simulink library "CTRL_LO_ST1_YAWTRQLATDIST"  (R2023b)
settings: Solver=VariableStepAuto  StartTime=0.0  StopTime=10.0  RelTol=1e-3
undefined symbols (not defined in the file): p_RadWhlDynFr_m, p_RadWhlDynRe_m
settings Model: Creator=blatak  LastModifiedBy=blatak

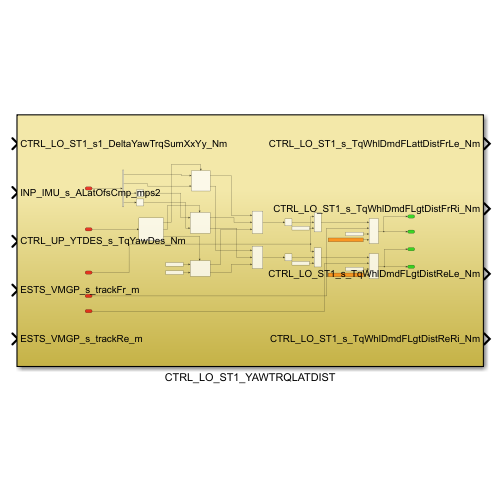
[thumbnail: Simulink's stored preview of the top-level diagram]
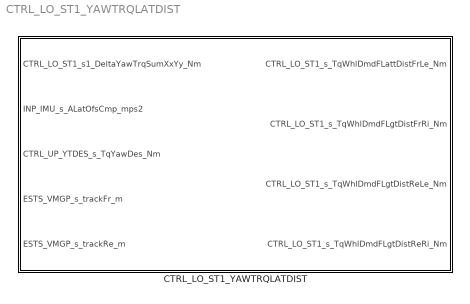
== system CTRL_LO_ST1_YAWTRQLATDIST ==
  CTRL_LO_ST1_YAWTRQLATDIST : Subsystem

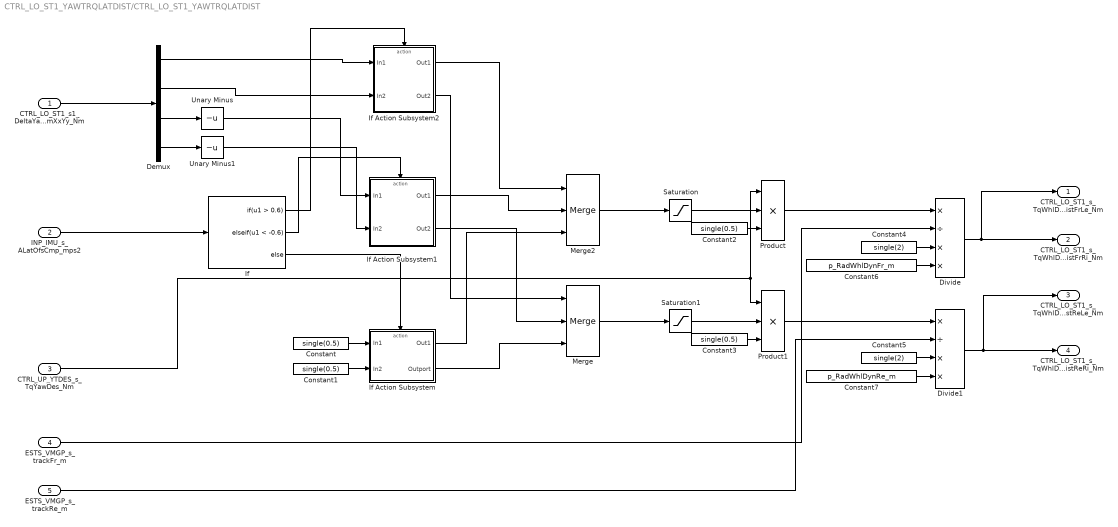
== system CTRL_LO_ST1_YAWTRQLATDIST/CTRL_LO_ST1_YAWTRQLATDIST ==
  CTRL_LO_ST1_s1_DeltaYawTrqSumXxYy_Nm : Inport
  INP_IMU_s_ALatOfsCmp_mps2 : Inport  Port=2
  CTRL_UP_YTDES_s_TqYawDes_Nm : Inport  Port=3
  ESTS_VMGP_s_trackFr_m : Inport  Port=4
  ESTS_VMGP_s_trackRe_m : Inport  Port=5
  Constant{,1..3} (4 alike) : Constant  Value=single(0.5)
  Constant4 : Constant  Value=single(2)
  Constant5 : Constant  Value=single(2)
  Constant6 : Constant  Value=p_RadWhlDynFr_m
  Constant7 : Constant  Value=p_RadWhlDynRe_m
  Demux : Demux
  Divide : Product  Inputs=*/**
  Divide1 : Product  Inputs=*/**
  If : If  IfExpression=u1 > 0.6  ElseIfExpressions=u1 < -0.6
  If Action Subsystem : Subsystem  TreatAsAtomicUnit=on
  If Action Subsystem1 : Subsystem  TreatAsAtomicUnit=on
  If Action Subsystem2 : Subsystem  TreatAsAtomicUnit=on
  Merge : Merge  Inputs=3
  Merge2 : Merge  Inputs=3
  Product : Product  Inputs=3
  Product1 : Product  Inputs=3
  Saturation : Saturate  UpperLimit=1  LowerLimit=0
  Saturation1 : Saturate
  Unary Minus : UnaryMinus
  Unary Minus1 : UnaryMinus
  CTRL_LO_ST1_s_TqWhlDmdFLattDistFrLe_Nm : Outport
  CTRL_LO_ST1_s_TqWhlDmdFLgtDistFrRi_Nm : Outport  Port=2
  CTRL_LO_ST1_s_TqWhlDmdFLgtDistReLe_Nm : Outport  Port=3
  CTRL_LO_ST1_s_TqWhlDmdFLgtDistReRi_Nm : Outport  Port=4
  wires:
  If Action Subsystem/2(Outport) -> Merge/3
  CTRL_UP_YTDES_s_TqYawDes_Nm/1 -> Product1/1, Product/1
  Unary Minus1/1 -> If Action Subsystem1/2(In2)
  Constant7/1 -> Divide1/4
  Constant4/1 -> Divide/3
  Divide1/1 -> CTRL_LO_ST1_s_TqWhlDmdFLgtDistReRi_Nm/1, CTRL_LO_ST1_s_TqWhlDmdFLgtDistReLe_Nm/1
  Demux/2 -> If Action Subsystem2/2(In2)
  Demux/4 -> Unary Minus1/1
  CTRL_LO_ST1_s1_DeltaYawTrqSumXxYy_Nm/1 -> Demux/1
  Constant5/1 -> Divide1/3
  Constant1/1 -> If Action Subsystem/2(In2)
  Saturation/1 -> Product/2
  Constant6/1 -> Divide/4
  If Action Subsystem2/2(Out2) -> Merge/1
  Constant2/1 -> Product/3
  If Action Subsystem1/2(Out2) -> Merge/2
  ESTS_VMGP_s_trackFr_m/1 -> Divide/2
  Saturation1/1 -> Product1/2
  Constant3/1 -> Product1/3
  Divide/1 -> CTRL_LO_ST1_s_TqWhlDmdFLgtDistFrRi_Nm/1, CTRL_LO_ST1_s_TqWhlDmdFLattDistFrLe_Nm/1
  Unary Minus/1 -> If Action Subsystem1/1(In1)
  If/1 -> If Action Subsystem2/Action
  ESTS_VMGP_s_trackRe_m/1 -> Divide1/2
  Merge/1 -> Saturation1/1
  If/3 -> If Action Subsystem/Action
  Product1/1 -> Divide1/1
  Merge2/1 -> Saturation/1
  If Action Subsystem1/1(Out1) -> Merge2/2
  Demux/3 -> Unary Minus/1
  If/2 -> If Action Subsystem1/Action
  Demux/1 -> If Action Subsystem2/1(In1)
  Product/1 -> Divide/1
  If Action Subsystem2/1(Out1) -> Merge2/1
  If Action Subsystem/1(Out1) -> Merge2/3
  Constant/1 -> If Action Subsystem/1(In1)
  INP_IMU_s_ALatOfsCmp_mps2/1 -> If/1

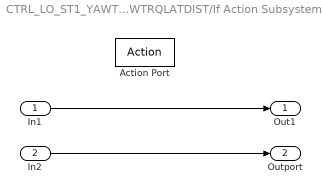
== system CTRL_LO_ST1_YAWTRQLATDIST/CTRL_LO_ST1_YAWTRQLATDIST/If Action Subsystem ==
  In1 : Inport
  In2 : Inport  Port=2
  Action Port : ActionPort  ActionPortLabel=else
  Out1 : Outport
  Outport : Outport  Port=2
  wires:
  In1/1 -> Out1/1
  In2/1 -> Outport/1

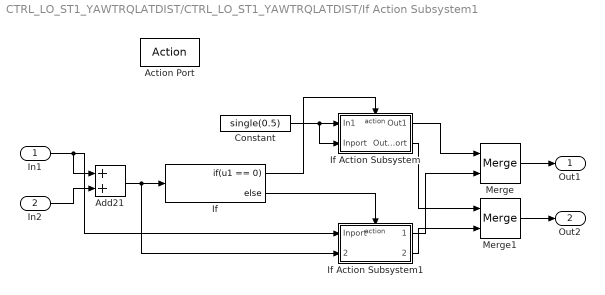
== system CTRL_LO_ST1_YAWTRQLATDIST/CTRL_LO_ST1_YAWTRQLATDIST/If Action Subsystem1 ==
  In1 : Inport
  In2 : Inport  Port=2
  Action Port : ActionPort  ActionPortLabel=elseif(u1 < -0.6)
  Add21 : Sum
  Constant : Constant  Value=single(0.5)
  If : If  IfExpression=u1 == 0
  If Action Subsystem : Subsystem  TreatAsAtomicUnit=on
  If Action Subsystem1 : Subsystem  TreatAsAtomicUnit=on
  Merge : Merge
  Merge1 : Merge
  Out1 : Outport
  Out2 : Outport  Port=2
  wires:
  If/1 -> If Action Subsystem/Action
  If/2 -> If Action Subsystem1/Action
  In1/1 -> If Action Subsystem1/1(Inport), Add21/1
  Constant/1 -> If Action Subsystem/1(In1), If Action Subsystem/2(Inport)
  Add21/1 -> If Action Subsystem1/2(Inport1), If/1
  If Action Subsystem1/1(Outport) -> Merge/2
  If Action Subsystem1/2(Outport1) -> Merge1/2
  If Action Subsystem/2(Outport) -> Merge1/1
  If Action Subsystem/1(Out1) -> Merge/1
  Merge1/1 -> Out2/1
  Merge/1 -> Out1/1
  In2/1 -> Add21/2

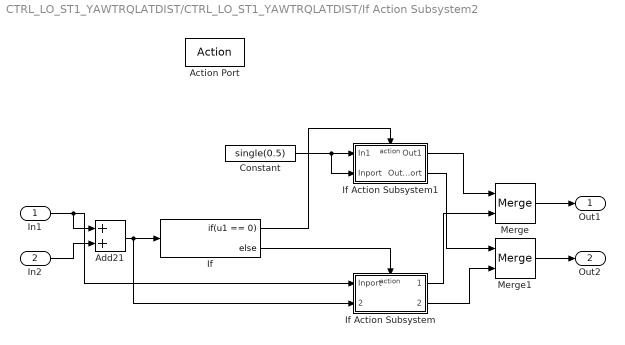
== system CTRL_LO_ST1_YAWTRQLATDIST/CTRL_LO_ST1_YAWTRQLATDIST/If Action Subsystem2 ==
  In1 : Inport
  In2 : Inport  Port=2
  Action Port : ActionPort  ActionPortLabel=if(u1 > 0.6)
  Add21 : Sum
  Constant : Constant  Value=single(0.5)
  If : If  IfExpression=u1 == 0
  If Action Subsystem : Subsystem  TreatAsAtomicUnit=on
  If Action Subsystem1 : Subsystem  TreatAsAtomicUnit=on
  Merge : Merge
  Merge1 : Merge
  Out1 : Outport
  Out2 : Outport  Port=2
  wires:
  If Action Subsystem1/1(Out1) -> Merge/1
  If/1 -> If Action Subsystem1/Action
  In2/1 -> Add21/2
  If Action Subsystem/1(Outport) -> Merge/2
  If Action Subsystem1/2(Outport) -> Merge1/1
  If Action Subsystem/2(Outport1) -> Merge1/2
  Merge1/1 -> Out2/1
  If/2 -> If Action Subsystem/Action
  Constant/1 -> If Action Subsystem1/1(In1), If Action Subsystem1/2(Inport)
  Add21/1 -> If Action Subsystem/2(Inport1), If/1
  In1/1 -> If Action Subsystem/1(Inport), Add21/1
  Merge/1 -> Out1/1

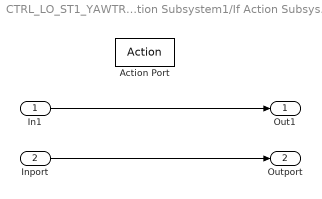
== system CTRL_LO_ST1_YAWTRQLATDIST/CTRL_LO_ST1_YAWTRQLATDIST/If Action Subsystem1/If Action Subsystem ==
  In1 : Inport
  Inport : Inport  Port=2
  Action Port : ActionPort  ActionPortLabel=if(u1 == 0)
  Out1 : Outport
  Outport : Outport  Port=2
  wires:
  In1/1 -> Out1/1
  Inport/1 -> Outport/1

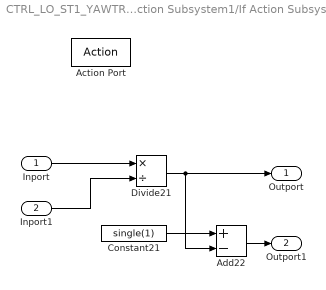
== system CTRL_LO_ST1_YAWTRQLATDIST/CTRL_LO_ST1_YAWTRQLATDIST/If Action Subsystem1/If Action Subsystem1 ==
  Inport : Inport
  Inport1 : Inport  Port=2
  Action Port : ActionPort  ActionPortLabel=else
  Add22 : Sum  Inputs=+-
  Constant21 : Constant  Value=single(1)
  Divide21 : Product  Inputs=*/
  Outport : Outport
  Outport1 : Outport  Port=2
  wires:
  Inport/1 -> Divide21/1
  Constant21/1 -> Add22/1
  Inport1/1 -> Divide21/2
  Add22/1 -> Outport1/1
  Divide21/1 -> Outport/1, Add22/2

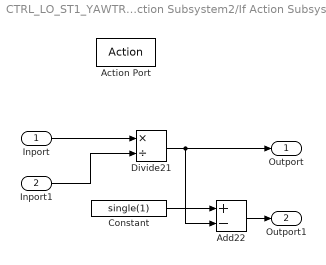
== system CTRL_LO_ST1_YAWTRQLATDIST/CTRL_LO_ST1_YAWTRQLATDIST/If Action Subsystem2/If Action Subsystem ==
  Inport : Inport
  Inport1 : Inport  Port=2
  Action Port : ActionPort  ActionPortLabel=else
  Add22 : Sum  Inputs=+-
  Constant : Constant  Value=single(1)
  Divide21 : Product  Inputs=*/
  Outport : Outport
  Outport1 : Outport  Port=2
  wires:
  Inport/1 -> Divide21/1
  Constant/1 -> Add22/1
  Inport1/1 -> Divide21/2
  Add22/1 -> Outport1/1
  Divide21/1 -> Outport/1, Add22/2

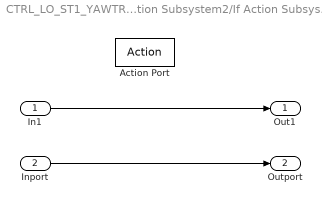
== system CTRL_LO_ST1_YAWTRQLATDIST/CTRL_LO_ST1_YAWTRQLATDIST/If Action Subsystem2/If Action Subsystem1 ==
  In1 : Inport
  Inport : Inport  Port=2
  Action Port : ActionPort  ActionPortLabel=if(u1 == 0)
  Out1 : Outport
  Outport : Outport  Port=2
  wires:
  In1/1 -> Out1/1
  Inport/1 -> Outport/1
